simulink model "pfb_core"  (R2012b)
settings: Solver=ode45  StartTime=0.0  StopTime=10.0  RelTol=1e-3
libraries: xbsIndex_r4 x656, casper_library_delays x1
(part 2 of 5)

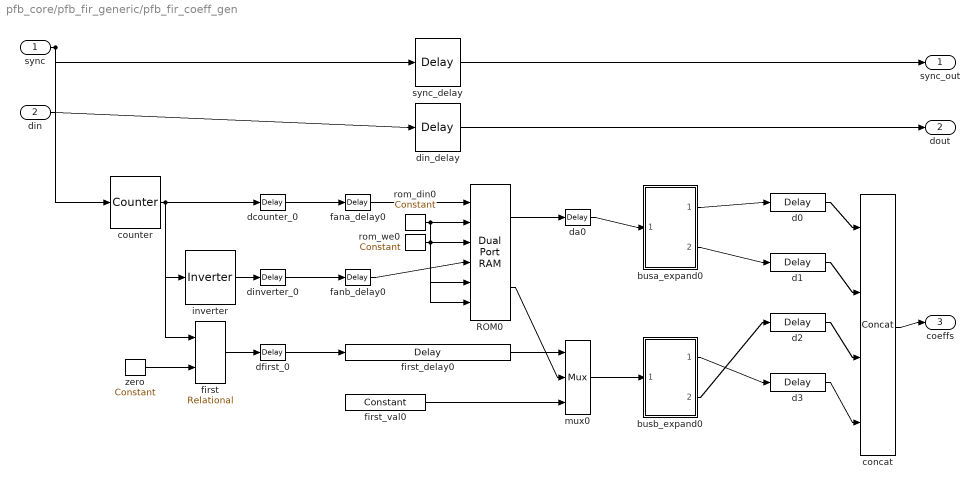
== system pfb_core/pfb_fir_generic/pfb_fir_coeff_gen ==
  sync : Inport
  din : Inport  Port=2
  ROM0 : xbsIndex_r4/Dual Port RAM  depth=2^(pfb_size-n_inputs)  initVector=[0 0 0 0 1 1 1 1 1 1 1 1 2 2 2 2 2 2 2 3 3 3 3 3 3 3 4 4 4 4 4 4 4 4 5 5 5 5 5 5 5 6 6 6 6 6 6 6 7 7 16773127 16773127 16773127 16773127 16773127 16773128 16773128 16773128 16773128 16773128 16773128 16773128 16773129 16773129 16773129 16773129 16773129 16773129 16773129 16773129 16773130 16773130 16773130 16773130 16773130 16773130 16773130 16773131 16773131 16773131 16773131 16773131 16773131 16773131 16773132 16773132 16773132 16773132 16773132 16773132 16773132 16773133 16773133 16773133 16773133 16773133 16773133 16773133 16773134 16773134 16773134 16773134 16773134 16773134 16773134 16773135 16773135 16773135 16773135 16773135 16773135 16773135 16773136 16773136 16773136 16773136 16773136 16773136 16773136 16773137 16773137 16773137 16773137 16773137 16773137 16773137 16773138 16773138 16773138 16773138 16773138 16773138 16773138 16773139 16773139 16773139 16773139 16773139 16773139 16773140 16773140 16773140 16773140 16773140 16773140 16773140 16773141 16773141 16773141 16769045 16769045 16769045 16769045 16769046 16769046 16769046 16769046 16769046 16769046 16769046 16769047 16769047 16769047 16769047 16769047 16769047 16769047 16769048 16769048 16769048 16769048 16769048 16769048 16769049 16769049 16769049 16769049 16769049 16769049 16769049 16769050 16769050 16769050 16769050 16769050 16769050 16769050 16769051 16769051 16769051 16769051 16769051 16769051 16769052 16769052 16769052 16769052 16769052 16769052 16769052 16769053 16769053 16769053 16769053 16769053 16769053 16769053 16769054 16769054 16769054 16769054 16769054 16769054 16769055 16769055 16769055 16769055 16769055 16769055 16769055 16769056 16769056 16769056 16769056 16769056 16769056 16769056 16769057 16769057 16769057 16769057 16769057 16769057 16769058 16769058 16769058 16769058 16769058 16769058 16769058 16769059 16769059 16769059 16769059 16769059 16769059 16764964 16764964 16764964 16764964 16764964 16764964 16764964 16764965 16764965 16764965 16764965 16764965 16764965 16764966 16764966 16764966 16764966 16764966 16764966 16764967 16764967 16764967 16764967 16764967 16764967 16764967 16764968 16764968 16764968 16764968 16764968 16764968 16764969 16764969 16764969 16764969 16764969 16764969 16764969 16764970 16764970 16764970 16764970 16764970 16764970 16764971 16764971 16764971 16764971 16764971 16764971 16764972 16764972 16764972 16764972 16764972 16764972 16764972 16764973 16764973 16764973 16764973 16764973 16764973 16764974 16764974 16764974 16764974 16764974 16764974 16764975 16764975 16764975 16764975 16764975 16764975 16764976 16764976 16764976 16764976 16764976 16764976 16764976 16764977 16764977 16764977 16764977 16764977 16764977 16764978 16764978 16764978 16764978 16764978 16760882 16760883 16760883 16760883 16760883 16760883 16760883 16760884 16760884 16760884 16760884 16760884 16760884 16760885 16760885 16760885 16760885 16760885 16760885 16760885 16760886 16760886 16760886 16760886 16760886 16760886 16760887 16760887 16760887 16760887 16760887 16760887 16760888 16760888 16760888 16760888 16760888 16760888 16760889 16760889 16760889 16760889 16760889 16760889 16760890 16760890 16760890 16760890 16760890 16760890 16760891 16760891 16760891 16760891 16760891 16760891 16760892 16760892 16760892 16760892 16760892 16760892 16760893 16760893 16760893 16760893 16760893 16760893 16760894 16760894 16760894 16760894 16760894 16760894 16760895 16760895 16760895 16760895 16760895 16760895 16760896 16760896 16760896 16760896 16760896 16760896 16760897 16760897 16760897 16760897 16760897 16760897 16756802 16756802 16756802 16756802 16756802 16756802 16756803 16756803 16756803 16756803 16756803 16756803 16756804 16756804 16756804 16756804 16756804 16756804 16756805 16756805 16756805 16756805 16756805 16756806 16756806 16756806 16756806 16756806 16756806 16756807 16756807 16756807 16756807 16756807 16756807 16756808 16756808 16756808 16756808 16756808 16756808 16756809 16756809 16756809 16756809 16756809 16756809 16756810 16756810 16756810 16756810 ...(+69369 chars)]  distributed_mem=Block RAM  init_a=0  init_b=0  rst_a=off  rst_b=off  en_a=off  en_b=off  latency=2  write_mode_A=Read After Write  write_mode_B=Read After Write  dbl_ovrd=off  optimize=Area  block_type=dpram
  busa_expand0 : Subsystem  AncestorBlock=casper_library_flow_control/bus_expand  mask(bus_expand){mode=divisions of equal size, outputNum=2, outputWidth=12, outputBinaryPt=0, outputArithmeticType=0, show_format=off, outputToWorkspace=off, variablePrefix=out, outputToModelAsWell=on}
      mask prompts: outputNum "Number of outputs:"; outputWidth "Output width:"; outputBinaryPt "Output binary point position:"; outputArithmeticType "Output arithmetic type (ufix=0, fix=1, bool=2):"; show_format "Print format string?"; outputToWorkspace "Output to workspace?"; variablePrefix "Variable name prefix:"; outputToModelAsWell "Output to model as well?"
      mask help:
      | Expands a 'bus' made using a bus_create or Xilinx
      | concat block.
      | The input will be divided into the specified number
      | of outputs with the specified arithmetic types.
      | Divisions are made from most significant bit.
      mask init: same as pfb_core/pfb_fir_generic/bus_expand
      settings: AttributesFormatString=2 outputs
      mask TypeOptions mode: divisions of equal size | divisions of arbitrary size
      mask Callback mode: bus_expand_callback();
      mask Callback outputWidth: bus_expand_callback();
      mask Callback outputToWorkspace: bus_expand_callback();
  busb_expand0 : Subsystem  AncestorBlock=casper_library_flow_control/bus_expand  mask(bus_expand){mode=divisions of equal size, outputNum=2, outputWidth=12, outputBinaryPt=0, outputArithmeticType=0, show_format=off, outputToWorkspace=off, variablePrefix=out, outputToModelAsWell=on}
      mask prompts: outputNum "Number of outputs:"; outputWidth "Output width:"; outputBinaryPt "Output binary point position:"; outputArithmeticType "Output arithmetic type (ufix=0, fix=1, bool=2):"; show_format "Print format string?"; outputToWorkspace "Output to workspace?"; variablePrefix "Variable name prefix:"; outputToModelAsWell "Output to model as well?"
      mask help:
      | Expands a 'bus' made using a bus_create or Xilinx
      | concat block.
      | The input will be divided into the specified number
      | of outputs with the specified arithmetic types.
      | Divisions are made from most significant bit.
      mask init: same as pfb_core/pfb_fir_generic/bus_expand
      settings: AttributesFormatString=2 outputs
      mask TypeOptions mode: divisions of equal size | divisions of arbitrary size
      mask Callback mode: bus_expand_callback();
      mask Callback outputWidth: bus_expand_callback();
      mask Callback outputToWorkspace: bus_expand_callback();
  concat : xbsIndex_r4/Concat  num_inputs=4  dbl_ovrd=off  block_type=concat
  counter : xbsIndex_r4/Counter  cnt_type=Free Running  cnt_to=Inf  operation=Up  start_count=0  cnt_by_val=1  arith_type=Unsigned  n_bits=13  bin_pt=0  load_pin=off  rst=on  en=off  explicit_period=on  period=1  dbl_ovrd=off  use_behavioral_HDL=off  implementation=Fabric  block_type=counter
  d0 : xbsIndex_r4/Delay  rst=off  infoeditControl=Selection of Reset will increase slice count due to use of real FFs and instead of SRLs  en=off  latency=6  dbl_ovrd=off  reg_retiming=on  block_type=delay
  d1 : xbsIndex_r4/Delay  rst=off  infoeditControl=Selection of Reset will increase slice count due to use of real FFs and instead of SRLs  en=off  latency=4  dbl_ovrd=off  reg_retiming=on  block_type=delay
  d2 : xbsIndex_r4/Delay  rst=off  infoeditControl=Selection of Reset will increase slice count due to use of real FFs and instead of SRLs  en=off  latency=2  dbl_ovrd=off  reg_retiming=on  block_type=delay
  d3 : xbsIndex_r4/Delay  rst=off  infoeditControl=Selection of Reset will increase slice count due to use of real FFs and instead of SRLs  en=off  latency=0  dbl_ovrd=off  reg_retiming=on  block_type=delay
  da0 : xbsIndex_r4/Delay  rst=off  infoeditControl=Selection of Reset will increase slice count due to use of real FFs and instead of SRLs  en=off  latency=1  dbl_ovrd=off  reg_retiming=on  block_type=delay
  dcounter_0 : xbsIndex_r4/Delay  rst=off  infoeditControl=Selection of Reset will increase slice count due to use of real FFs and instead of SRLs  en=off  latency=1  dbl_ovrd=off  reg_retiming=off  block_type=delay
  dfirst_0 : xbsIndex_r4/Delay  rst=off  infoeditControl=Selection of Reset will increase slice count due to use of real FFs and instead of SRLs  en=off  latency=1  dbl_ovrd=off  reg_retiming=off  block_type=delay
  din_delay : xbsIndex_r4/Delay  rst=off  infoeditControl=Selection of Reset will increase slice count due to use of real FFs and instead of SRLs  en=off  latency=5  dbl_ovrd=off  reg_retiming=on  block_type=delay
  dinverter_0 : xbsIndex_r4/Delay  rst=off  infoeditControl=Selection of Reset will increase slice count due to use of real FFs and instead of SRLs  en=off  latency=1  dbl_ovrd=off  reg_retiming=off  block_type=delay
  fana_delay0 : xbsIndex_r4/Delay  rst=off  infoeditControl=Selection of Reset will increase slice count due to use of real FFs and instead of SRLs  en=off  latency=1  dbl_ovrd=off  reg_retiming=off  block_type=delay
  fanb_delay0 : xbsIndex_r4/Delay  rst=off  infoeditControl=Selection of Reset will increase slice count due to use of real FFs and instead of SRLs  en=off  latency=1  dbl_ovrd=off  reg_retiming=off  block_type=delay
  first : xbsIndex_r4/Relational  mode=a=b  en=off  latency=0  dbl_ovrd=off  block_type=relational
  first_delay0 : xbsIndex_r4/Delay  rst=off  infoeditControl=Selection of Reset will increase slice count due to use of real FFs and instead of SRLs  en=off  latency=3  dbl_ovrd=off  reg_retiming=off  block_type=delay
  first_val0 : xbsIndex_r4/Constant  const=2047  gui_display_data_type=Fixed-point  arith_type=Unsigned  n_bits=24  bin_pt=0  preci_type=Single  exp_width=8  frac_width=24  explicit_period=on  period=1  equ=P=C  opselect=C  inp2=PCIN>>17  opr=+  inp1=P  carry=CIN  dbl_ovrd=off  block_type=constant
  inverter : xbsIndex_r4/Inverter  en=off  latency=1  dbl_ovrd=off  block_type=inv
  mux0 : xbsIndex_r4/Mux  inputs=2  en=off  latency=1  precision=Full  arith_type=Unsigned  n_bits=16  bin_pt=14  quantization=Truncate  overflow=Wrap  dbl_ovrd=off  block_type=mux
  rom_din0 : xbsIndex_r4/Constant  const=0  gui_display_data_type=Fixed-point  arith_type=Unsigned  n_bits=24  bin_pt=0  preci_type=Single  exp_width=8  frac_width=24  explicit_period=on  period=1  equ=P=C  opselect=C  inp2=PCIN>>17  opr=+  inp1=P  carry=CIN  dbl_ovrd=off  block_type=constant
  rom_we0 : xbsIndex_r4/Constant  const=0  gui_display_data_type=Fixed-point  arith_type=Boolean  n_bits=16  bin_pt=14  preci_type=Single  exp_width=8  frac_width=24  explicit_period=on  period=1  equ=P=C  opselect=C  inp2=PCIN>>17  opr=+  inp1=P  carry=CIN  dbl_ovrd=off  block_type=constant
  sync_delay : xbsIndex_r4/Delay  rst=off  infoeditControl=Selection of Reset will increase slice count due to use of real FFs and instead of SRLs  en=off  latency=5  dbl_ovrd=off  reg_retiming=on  block_type=delay
  zero : xbsIndex_r4/Constant  const=0  gui_display_data_type=Fixed-point  arith_type=Unsigned  n_bits=13  bin_pt=0  preci_type=Single  exp_width=8  frac_width=24  explicit_period=on  period=1  equ=P=C  opselect=C  inp2=PCIN>>17  opr=+  inp1=P  carry=CIN  dbl_ovrd=off  block_type=constant
  sync_out : Outport
  dout : Outport  Port=2
  coeffs : Outport  Port=3
  wires:
  busb_expand0/1(msb_out2) -> d3/1
  busb_expand0/2(lsb_out1) -> d2/1
  busa_expand0/2(lsb_out1) -> d1/1
  busa_expand0/1(msb_out2) -> d0/1
  d3/1 -> concat/4
  d2/1 -> concat/3
  d1/1 -> concat/2
  d0/1 -> concat/1
  concat/1 -> coeffs/1
  mux0/1 -> busb_expand0/1(bus_in)
  da0/1 -> busa_expand0/1(bus_in)
  first_val0/1 -> mux0/3
  ROM0/2 -> mux0/2
  first_delay0/1 -> mux0/1
  ROM0/1 -> da0/1
  rom_we0/1 -> ROM0/6, ROM0/3
  rom_din0/1 -> ROM0/5, ROM0/2
  fanb_delay0/1 -> ROM0/4
  fana_delay0/1 -> ROM0/1
  dfirst_0/1 -> first_delay0/1
  dinverter_0/1 -> fanb_delay0/1
  dcounter_0/1 -> fana_delay0/1
  first/1 -> dfirst_0/1
  inverter/1 -> dinverter_0/1
  zero/1 -> first/2
  counter/1 -> dcounter_0/1, first/1, inverter/1
  din_delay/1 -> dout/1
  din/1 -> din_delay/1
  sync_delay/1 -> sync_out/1
  sync/1 -> counter/1, sync_delay/1
